simulink model "DDS"  (R2018b)
settings: Solver=VariableStepAuto  StartTime=0.0  StopTime=10.0  RelTol=1e-3
settings Model: Creator=Administrator  LastModifiedBy=Administrator

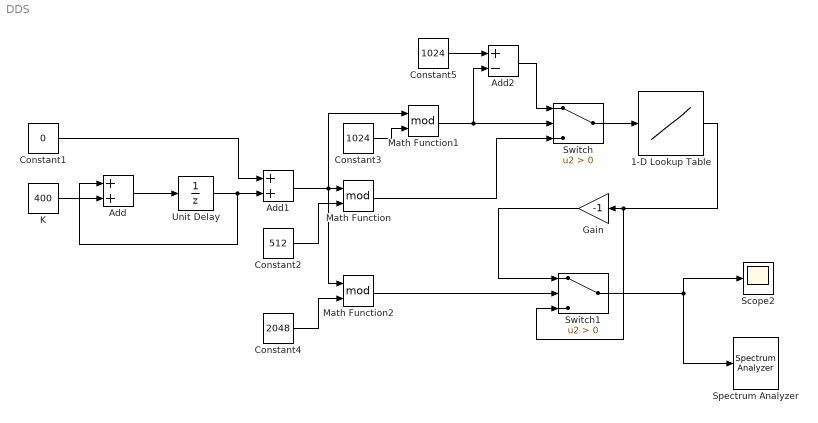
== system DDS ==
  1-D Lookup Table : Lookup_n-D  NumberOfTableDimensions=1  BreakpointsForDimension1=[0:512]  Table=sin([0:512]/1024*pi)  InternalRulePriority=Speed  RndMeth=Simplest  InputSameDT=on
  Add : Sum
  Add1 : Sum
  Add2 : Sum  Inputs=+-
  Constant1 : Constant  Value=0
  Constant2 : Constant  Value=512
  Constant3 : Constant  Value=1024
  Constant4 : Constant  Value=2048
  Constant5 : Constant  Value=1024
  Gain : Gain  Gain=-1
  K : Constant  Value=400
  Math Function : Math  Operator=mod  SaturateOnIntegerOverflow=on
  Math Function1 : Math  Operator=mod  SaturateOnIntegerOverflow=on
  Math Function2 : Math  Operator=mod  SaturateOnIntegerOverflow=on
  Scope2 : Scope
  Spectrum Analyzer : SpectrumAnalyzer
  Switch : Switch  Criteria=u2 > Threshold
  Switch1 : Switch  Criteria=u2 > Threshold
  Unit Delay : UnitDelay  SampleTime=-1
  wires:
  K/1 -> Add/2
  Add/1 -> Unit Delay/1
  Unit Delay/1 -> Add/1, Add1/2
  Constant1/1 -> Add1/1
  Add1/1 -> Math Function1/1, Math Function/1, Math Function2/1
  Constant2/1 -> Math Function/2
  Constant4/1 -> Math Function2/2
  Constant3/1 -> Math Function1/2
  Constant5/1 -> Add2/1
  Math Function1/1 -> Switch/2, Add2/2
  Switch/1 -> 1-D Lookup Table/1
  Add2/1 -> Switch/1
  Math Function/1 -> Switch/3
  Math Function2/1 -> Switch1/2
  Gain/1 -> Switch1/1
  1-D Lookup Table/1 -> Switch1/3, Gain/1
  Switch1/1 -> Spectrum Analyzer/1, Scope2/1
